simulink model "APS"  (R2020a)
settings: Solver=FixedStepAuto  StartTime=0.0  StopTime=15  FixedStep=0.01  RelTol=1e-3  EnableMultiTasking=on
libraries: embdlinuxlib x3, raspberrypiBasiclib x3
settings Model: SimulationMode=external  Creator=hps  LastModifiedBy=郑亮
settings SolverCC: PositivePriorityOrder=on  AutoInsertRateTranBlk=on
settings DataIOCC: ReturnWorkspaceOutputs=off
settings OptimizationCC: EnhancedBackFolding=on  PassReuseOutputArgsAs=Individual arguments  MaxStackSize=64  OptimizeBlockOrder=speed  DifferentSizesBufferReuse=on  OptimizationCustomize=off  EfficientTunableParamExpr=on
settings DebuggingCC: ParameterTunabilityLossMsg=error  ArithmeticOperatorsInVariantConditions=warning
settings HardwareCC: ProdBitPerPointer=32  ProdBitPerSizeT=32  ProdBitPerPtrDiffT=32  ProdLargestAtomicInteger=Long  ProdLargestAtomicFloat=Double  ProdWordSize=32  ProdHWDeviceType=ARM Compatible->ARM Cortex
settings SFSimCC: MATLABDynamicMemAlloc=off  CustomCodeUndefinedFunction=UseInterfaceOnly
settings RTWCC: SystemTargetFile=ert.tlc  HardwareBoard=Raspberry Pi  TemplateMakefile=ert_default_tmf  GenerateReport=on  Toolchain=GNU GCC Raspberry Pi  BuildConfiguration=Faster Runs  IncludeHyperlinkInReport=on  LaunchReport=on  GenerateTraceInfo=on  GenerateTraceReport=on  GenerateTraceReportSl=on  GenerateTraceReportSf=on  GenerateTraceReportEml=on
settings CodeAppCC: ForceParamTrailComments=on  IgnoreCustomStorageClasses=off  OperatorAnnotations=on  SimulinkDataObjDesc=on  SFDataObjDesc=on  InsertBlockDesc=on
settings ERTTargetCC: SupportContinuousTime=on  SupportVariableSizeSignals=on  ExtModeMexArgs='192.168.43.221' 0 12705

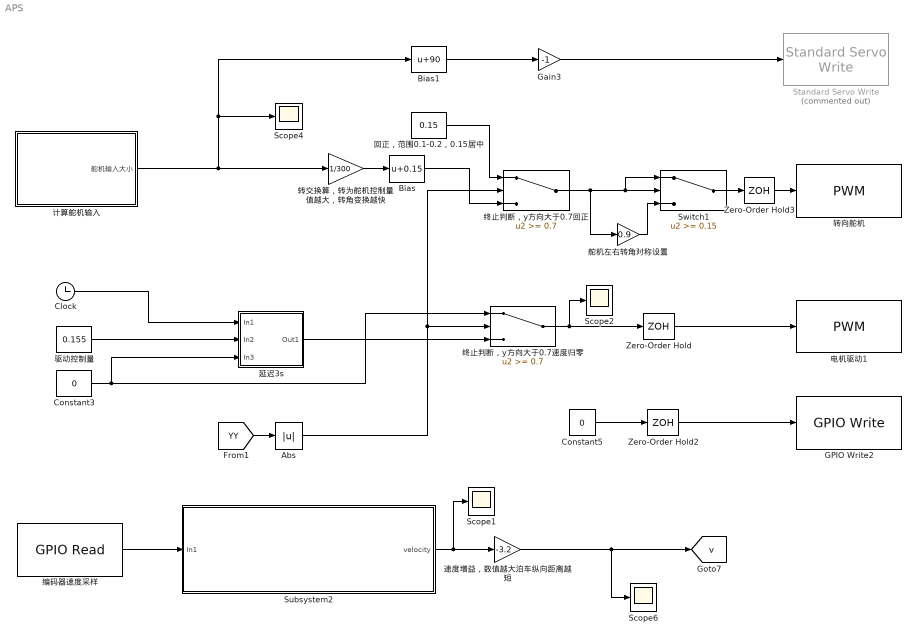
== system APS ==
  Abs : Abs
  Bias : Bias  Bias=0.15
  Bias1 : Bias  Bias=90
  Clock : Clock
  Constant3 : Constant  Value=0
  Constant5 : Constant  Value=0
  GPIO Write2 : embdlinuxlib/GPIO Write  board=Pi 3 Model B+  gpio=27  direction=Output  blockPlatform=Raspberry Pi
      settings: SourceProductBaseCode=SC_BEAGLEBONE_BLUE,RASPPI
  Gain3 : Gain  Gain=-1
  Scope{1..2,4,6} (4 alike) : Scope
  Standard Servo Write : raspberrypiBasiclib/Standard Servo Write  Commented=on  board=Pi 3 Model B+  Pin_=21  MinPulseDuration=1000e-6  MaxPulseDuration=2000e-6  blockPlatform=Raspberry Pi
      settings: SourceProductBaseCode=RASPPI
  Subsystem2 : Subsystem
  Switch1 : Switch  Threshold=0.15
  Zero-Order Hold : ZeroOrderHold  SampleTime=-1
  Zero-Order Hold2 : ZeroOrderHold  SampleTime=-1
  Zero-Order Hold3 : ZeroOrderHold  SampleTime=-1
  回正，范围0.1-0.2，0.15居中 : Constant  Value=0.15
  延迟3s : Subsystem
  电机驱动1 : raspberrypiBasiclib/PWM  board=Pi 3 Model B+  Pin_=17  Frequency=8000  blockPlatform=Raspberry Pi
      settings: SourceProductBaseCode=RASPPI
  终止判断，y方向大于0.7回正 : Switch  Threshold=0.7
  终止判断，y方向大于0.7速度归零 : Switch  Threshold=0.7
  编码器速度采样 : embdlinuxlib/GPIO Read  board=Pi 3 Model B+  gpio=14  internalResistor=Off  sampleTime=0.01  direction=Input  blockPlatform=Raspberry Pi
      settings: SourceProductBaseCode=SC_BEAGLEBONE_BLUE,RASPPI
  舵机左右转角对称设置 : Gain  Gain=0.9
  计算舵机输入 : Subsystem
  "转交换算，转为舵机控制量 值越大，转角变换越快 " : Gain  Gain=1/300
  转向舵机 : raspberrypiBasiclib/PWM  board=Pi 3 Model B  Pin_=21  Frequency=100  blockPlatform=Raspberry Pi
      settings: SourceProductBaseCode=RASPPI
  速度增益，数值越大泊车纵向距离越短 : Gain  Gain=-3.2
  驱动控制量 : Constant  Value=0.155
  tag scope: v=global
  wires:
  Constant3/1 -> 延迟3s/3(In3), 终止判断，y方向大于0.7速度归零/1
  Clock/1 -> 延迟3s/1(In1)
  [YY] -> Abs/1
  Abs/1 -> 终止判断，y方向大于0.7回正/2, 终止判断，y方向大于0.7速度归零/2
  驱动控制量/1 -> 延迟3s/2(In2)
  延迟3s/1(Out1) -> 终止判断，y方向大于0.7速度归零/3
  计算舵机输入/1(舵机输入大小) -> Scope4/1, Bias1/1, "转交换算，转为舵机控制量 值越大，转角变换越快 "/1
  终止判断，y方向大于0.7速度归零/1 -> Zero-Order Hold/1, Scope2/1
  Zero-Order Hold3/1 -> 转向舵机/1
  Constant5/1 -> Zero-Order Hold2/1
  Zero-Order Hold/1 -> 电机驱动1/1
  Zero-Order Hold2/1 -> GPIO Write2/1
  Gain3/1 -> Standard Servo Write/1
  "转交换算，转为舵机控制量 值越大，转角变换越快 "/1 -> Bias/1
  Bias/1 -> 终止判断，y方向大于0.7回正/3
  Bias1/1 -> Gain3/1
  速度增益，数值越大泊车纵向距离越短/1 -> Scope6/1, [v]
  编码器速度采样/1 -> Subsystem2/1(In1)
  Subsystem2/1("velocity ") -> Scope1/1, 速度增益，数值越大泊车纵向距离越短/1
  回正，范围0.1-0.2，0.15居中/1 -> 终止判断，y方向大于0.7回正/1
  终止判断，y方向大于0.7回正/1 -> 舵机左右转角对称设置/1, Switch1/1, Switch1/2
  舵机左右转角对称设置/1 -> Switch1/3
  Switch1/1 -> Zero-Order Hold3/1

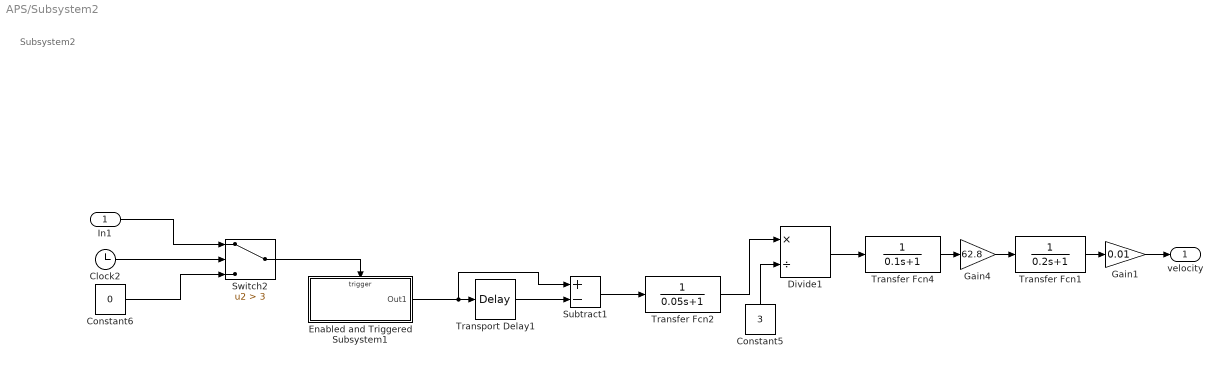
== system APS/Subsystem2 ==
  note: Subsystem2
  In1 : Inport
  Clock2 : Clock
  Constant5 : Constant  Value=3
  Constant6 : Constant  Value=0
  Divide1 : Product  Inputs=*/
  Enabled and Triggered Subsystem1 : Subsystem  TreatAsAtomicUnit=on
  Gain1 : Gain  Gain=0.01
  Gain4 : Gain  Gain=62.8
  Subtract1 : Sum  Inputs=+-
  Switch2 : Switch  Criteria=u2 > Threshold  Threshold=3
  Transfer Fcn1 : TransferFcn  Denominator=[0.2 1]
  Transfer Fcn2 : TransferFcn  Denominator=[0.05 1]
  Transfer Fcn4 : TransferFcn  Denominator=[0.1 1]
  Transport Delay1 : TransportDelay  DelayTime=0.5
  "velocity " : Outport  VectorParamsAs1DForOutWhenUnconnected=off
  wires:
  Constant6/1 -> Switch2/3
  Transport Delay1/1 -> Subtract1/2
  Enabled and Triggered Subsystem1/1(Out1) -> Subtract1/1, Transport Delay1/1
  Switch2/1 -> Enabled and Triggered Subsystem1/Trigger
  Transfer Fcn1/1 -> Gain1/1
  Subtract1/1 -> Transfer Fcn2/1
  Constant5/1 -> Divide1/2
  Clock2/1 -> Switch2/2
  In1/1 -> Switch2/1
  Transfer Fcn2/1 -> Divide1/1
  Gain4/1 -> Transfer Fcn1/1
  Divide1/1 -> Transfer Fcn4/1
  Transfer Fcn4/1 -> Gain4/1
  Gain1/1 -> "velocity "/1

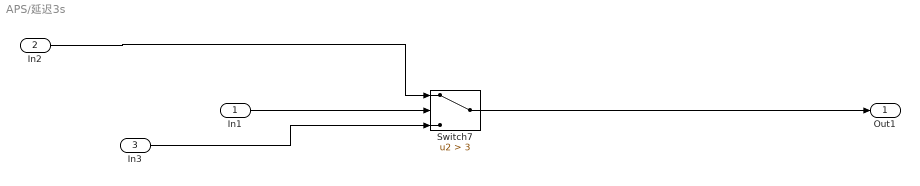
== system APS/延迟3s ==
  In1 : Inport
  In2 : Inport  Port=2
  In3 : Inport  Port=3
  Switch7 : Switch  Criteria=u2 > Threshold  Threshold=3
  Out1 : Outport  VectorParamsAs1DForOutWhenUnconnected=off
  wires:
  In3/1 -> Switch7/3
  In1/1 -> Switch7/2
  In2/1 -> Switch7/1
  Switch7/1 -> Out1/1

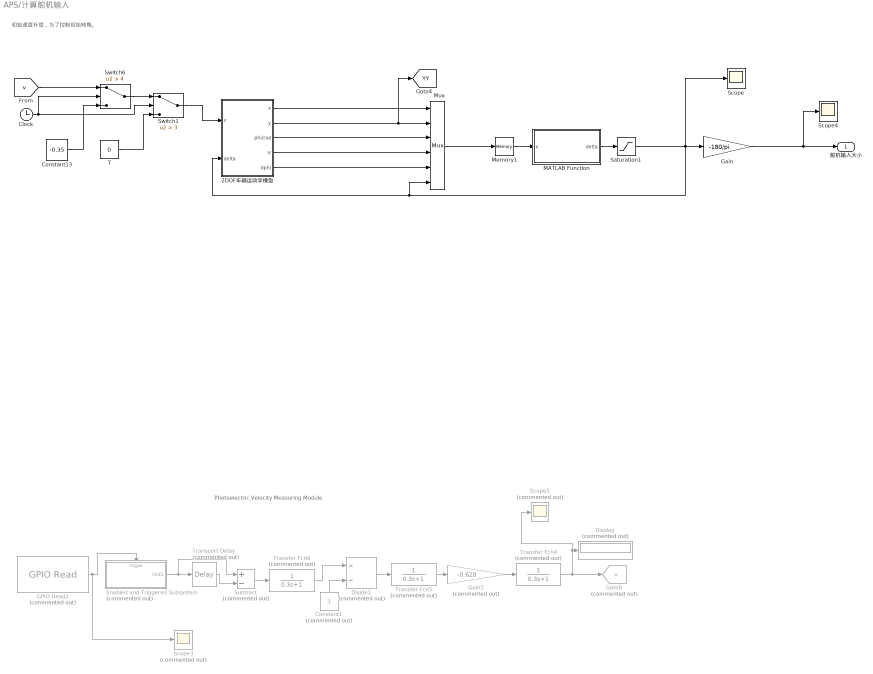
== system APS/计算舵机输入 ==
  note: 初始速度补偿，为了控制初始转角。
  note: Photoelectric Velocity Measuring Module
  2DOF车辆运动学模型 : Subsystem
  Clock : Clock
  Constant1 : Constant  Commented=on  Value=3
  Constant13 : Constant  Value=-0.35
  Display : Display  Commented=on
  Divide1 : Product  Commented=on  Inputs=*/
  Enabled and Triggered Subsystem : Subsystem  Commented=on  TreatAsAtomicUnit=on
  GPIO Read2 : embdlinuxlib/GPIO Read  Commented=on  board=Pi 3 Model B+  gpio=20  internalResistor=Off  sampleTime=0.01  direction=Input  blockPlatform=Raspberry Pi
      settings: SourceProductBaseCode=SC_BEAGLEBONE_BLUE,RASPPI
  Gain : Gain  Gain=-180/pi
  Gain2 : Gain  Commented=on  Gain=-0.628
  Goto8 : Goto  Commented=on  GotoTag=v  TagVisibility=global
  MATLAB Function : MATLAB Function  TreatAsAtomicUnit=on
  Memory1 : Memory
  Mux : Mux  Inputs=6
  Saturation1 : Saturate
  Scope : Scope
  Scope3 : Scope  Commented=on
  Scope4 : Scope
  Scope5 : Scope  Commented=on
  Subtract : Sum  Commented=on  Inputs=+-
  Switch1 : Switch  Criteria=u2 > Threshold  Threshold=3
  Switch6 : Switch  Criteria=u2 > Threshold  Threshold=4
  T : Constant  Value=0
  Transfer Fcn4 : TransferFcn  Commented=on  Denominator=[0.3 1]
  Transfer Fcn5 : TransferFcn  Commented=on  Denominator=[0.3 1]
  Transfer Fcn6 : TransferFcn  Commented=on  Denominator=[0.3 1]
  Transport Delay : TransportDelay  Commented=on  DelayTime=0.5
  舵机输入大小 : Outport  VectorParamsAs1DForOutWhenUnconnected=off
  tag scope: YY=global
  wires:
  Memory1/1 -> MATLAB Function/1(x)
  MATLAB Function/1(delta) -> Saturation1/1
  2DOF车辆运动学模型/5(dphi) -> Mux/5
  Switch1/1 -> 2DOF车辆运动学模型/1(v)
  2DOF车辆运动学模型/4(V) -> Mux/4
  2DOF车辆运动学模型/1(x) -> Mux/1
  2DOF车辆运动学模型/3(phi/rad) -> Mux/3
  Saturation1/1 -> Scope/1, Gain/1, Mux/6, 2DOF车辆运动学模型/2(delta)
  [v] -> Switch6/1
  2DOF车辆运动学模型/2(y) -> Mux/2, [YY]
  Mux/1 -> Memory1/1
  Transport Delay/1 -> Subtract/2
  Enabled and Triggered Subsystem/1(Out1) -> Transport Delay/1, Subtract/1
  Transfer Fcn4/1 -> Goto8/1, Scope5/1, Display/1
  Transfer Fcn5/1 -> Gain2/1
  Gain2/1 -> Transfer Fcn4/1
  Transfer Fcn6/1 -> Divide1/1
  Constant1/1 -> Divide1/2
  Subtract/1 -> Transfer Fcn6/1
  Divide1/1 -> Transfer Fcn5/1
  GPIO Read2/1 -> Scope3/1, Enabled and Triggered Subsystem/Trigger
  Gain/1 -> Scope4/1, 舵机输入大小/1
  Switch6/1 -> Switch1/1
  T/1 -> Switch1/3
  Constant13/1 -> Switch6/3
  Clock/1 -> Switch6/2, Switch1/2

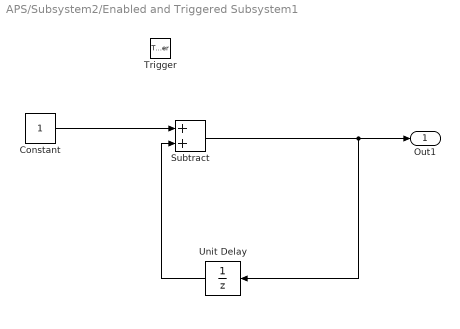
== system APS/Subsystem2/Enabled and Triggered Subsystem1 ==
  Trigger : TriggerPort  TriggerType=falling  VariantControl=Variant
  Constant : Constant
  Subtract : Sum
  Unit Delay : UnitDelay  SampleTime=-1  HasFrameUpgradeWarning=on
  Out1 : Outport  VectorParamsAs1DForOutWhenUnconnected=off
  wires:
  Constant/1 -> Subtract/1
  Subtract/1 -> Unit Delay/1, Out1/1
  Unit Delay/1 -> Subtract/2

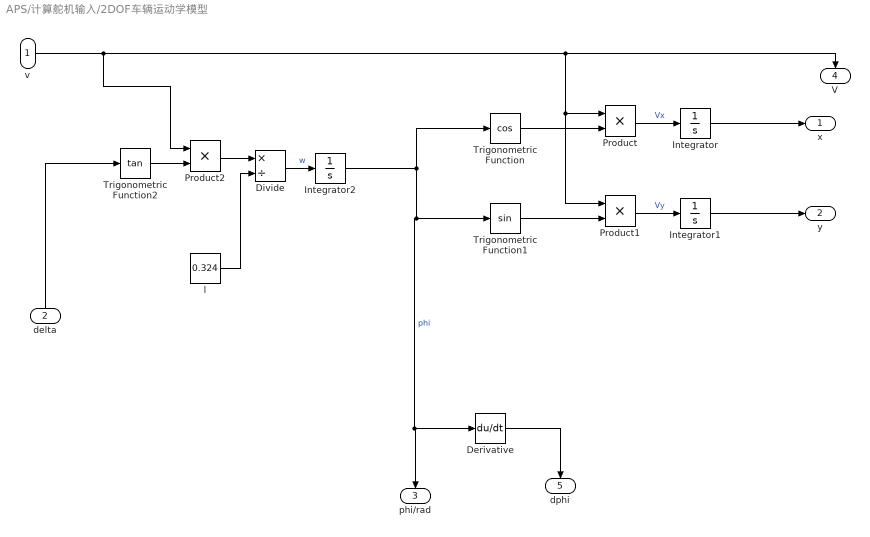
== system APS/计算舵机输入/2DOF车辆运动学模型 ==
  v : Inport
  delta : Inport  Port=2
  Derivative : Derivative
  Divide : Product  Inputs=*/
  Integrator : Integrator
  Integrator1 : Integrator
  Integrator2 : Integrator
  Product : Product
  Product1 : Product
  Product2 : Product
  Trigonometric Function : Trigonometry  Operator=cos
  Trigonometric Function1 : Trigonometry
  Trigonometric Function2 : Trigonometry  Operator=tan
  l : Constant  Value=0.324
  x : Outport  VectorParamsAs1DForOutWhenUnconnected=off
  y : Outport  Port=2  VectorParamsAs1DForOutWhenUnconnected=off
  phi/rad : Outport  Port=3  VectorParamsAs1DForOutWhenUnconnected=off
  V : Outport  Port=4  VectorParamsAs1DForOutWhenUnconnected=off
  dphi : Outport  Port=5  VectorParamsAs1DForOutWhenUnconnected=off
  wires:
  Derivative/1 -> dphi/1
  v/1 -> Product2/1, Product/1, Product1/1, V/1
  delta/1 -> Trigonometric Function2/1
  Integrator/1 -> x/1
  Integrator2/1 -> phi/rad/1, Derivative/1, Trigonometric Function1/1, Trigonometric Function/1  "phi"
  Integrator1/1 -> y/1
  Product1/1 -> Integrator1/1  "Vy"
  Trigonometric Function1/1 -> Product1/2
  Divide/1 -> Integrator2/1  "w"
  Product2/1 -> Divide/1
  Trigonometric Function/1 -> Product/2
  Trigonometric Function2/1 -> Product2/2
  l/1 -> Divide/2
  Product/1 -> Integrator/1  "Vx"

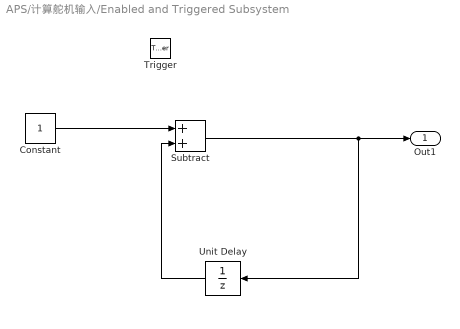
== system APS/计算舵机输入/Enabled and Triggered Subsystem ==
  Trigger : TriggerPort  TriggerType=falling  VariantControl=Variant
  Constant : Constant
  Subtract : Sum
  Unit Delay : UnitDelay  SampleTime=-1  HasFrameUpgradeWarning=on
  Out1 : Outport  VectorParamsAs1DForOutWhenUnconnected=off
  wires:
  Constant/1 -> Subtract/1
  Subtract/1 -> Unit Delay/1, Out1/1
  Unit Delay/1 -> Subtract/2

== matlab function APS/计算舵机输入/MATLAB Function ==
  data: x input; delta output
function delta = fcn(x)

    Nx = 3;%状态量的个数
    Nu = 2;%控制量的个数
    Ny = 2; %输出量的个数
    Np = 20;%预测步长
    Nc = 5;%控制步长
    Row = 1000;%松弛因子

    u = zeros(6,1);
    u = x;
    U = [0;u(6)];
    
    t_d =u(3);
    vd1=u(4);
    vd2=u(6); 
    
    kesi=zeros(Nx+Nu,1);  
    kesi(1)=u(1);
    kesi(2)=u(2);
    kesi(3)=u(3);   % 角度单位要一致！！！！！    
    kesi(4)=U(1);
    kesi(5)=U(2); 

    T=0.04;
    L = 0.324;
    
    u_piao=zeros(Nu,1);
    
    Q = zeros(2*Np,2*Np);
   for i=1:1:2*Np
       for j=1:1:2*Np
           if i==j
               if mod(i,2)==0
                   Q(i,j) = 1;
               else
                   Q(i,j) = 10;
               end
           else 
               Q(i,j)= 0;               
           end
       end 
   end 

    R = 10*eye(Nu*Nc);
    
    a=[1    0   -vd1*sin(t_d)*T;
       0    1   vd1*cos(t_d)*T;
       0    0   1;];
    b=[cos(t_d)*T            0;
       sin(t_d)*T            0;
       tan(vd2)*T/L      vd1*T/(cos(vd2)^2);];

    A = zeros(5,5);
    B = zeros(5,2);
    A(1:3,1:3)=a;
    A(1:3,4:5)=b;
    A(4:5,4:5)=eye(Nu);
    
    B(1:3,1:2)=b;
    B(4:5,1:2)=eye(Nu);

    C=[0 1 0 0 0;0 0 1 0 0;];

%% 计算偏差
    d_k=zeros(Nx,1);%计算偏差
    state_k1=zeros(Nx,1);%预测的下一时刻状态量，用于计算偏差
    state_k1(1,1)=u(1)+T*u(4)*cos(t_d);
    state_k1(2,1)=u(2)+T*u(4)*sin(t_d);
    state_k1(3,1)=t_d+T*u(5);
    d_k=state_k1-a*kesi(1:3,1)-b*kesi(4:5,1);
    d_piao_k=zeros(Nx+Nu,1);
    d_piao_k(1:3,1)=d_k;
    d_piao_k(4,1)=0;
    d_piao_k(5,1)=0;
    
    PHI = zeros(100,1);
    GAMMA = zeros(40,100);

    for p=1:1:Np
        PHI((5*(p-1)+1):(5*p),1)=d_piao_k;
        for q=1:1:Np
            if q<=p
                GAMMA((2*(p-1)+1):2*p,(5*(q-1)+1):5*q)=C*A^(p-q);
            else 
                GAMMA((2*(p-1)+1):2*p,(5*(q-1)+1):5*q)=zeros(Ny,Nx+Nu);
            end 
        end
    end
 
    PSI = zeros(40,5);
    THETA = zeros(40,10);
    for j=1:1:Np
       PSI((2*(j-1)+1):2*j,1:5)=C*A^j;
        for k=1:1:Nc
            if k<=j
                THETA((2*(j-1)+1):2*j,(2*(k-1)+1):2*k) = C*A^(j-k)*B;
            else 
                THETA((2*(j-1)+1):2*j,(2*(k-1)+1):2*k) = zeros(Ny,Nu);
            end
        end
    end    

    H = zeros(10,10);
    H(1:10,1:10)=THETA'*Q*THETA+R;
%     H(1:10,11)=zeros(Nu*Nc,1);
%     H(11,1:10)=zeros(1,Nu*Nc);
%     H(11,11)=Row;
        
%% 参考轨迹生成
    X_predict=zeros(Np,1);%用于保存预测时域内的纵向位置信息，这是计算期望轨迹的基础
    phi_ref=zeros(Np,1);%用于保存预测时域内的期望轨迹
    Y_ref=zeros(Np,1);%用于保存预测时域内的期望轨迹    
    Yita_ref=zeros(2*Np,1);
    error_1=zeros(Nx*Np,1);
    for p=1:1:Np
    %x=8 y=2.5
          X_predict(p,1)=u(1)+u(4)*cos(t_d)*p*T;
%           Y_ref(p,1)= 0.2;
%           phi_ref(p,1)=0;       
          Y_ref(p,1)=0.7/2*X_predict(p,1)-(-0.7/(2*pi))*sin((2*pi*X_predict(p,1))/(-2));
          phi_ref(p,1)=atan(0.7/2-(-0.7/(2*pi))*cos(2*pi*X_predict(p,1)/(-2))*2*pi/(-2)); 
          if Y_ref(p,1)<-0.7
             Y_ref(p,1)= -0.7;
             phi_ref(p,1) = 0;
          end
          Yita_ref((2*(p-1)+1):2*p,1)=[Y_ref(p,1);phi_ref(p,1)];
    end
    
    error_1=Yita_ref-PSI*kesi-GAMMA*PHI; %求偏差
    f=zeros(1,10);
%     f(1,1:10)=-2*error_1'*Q*THETA;
    f(1,1:10)=-2*error_1'*Q*THETA;
%     f(1,11)=0;
    f = f';
    
 %% 以下为约束生成区域
 %不等式约束
    A_t=zeros(Nc,Nc);
    for p=1:1:Nc
        for q=1:1:Nc
            if q<=p 
                A_t(p,q)=1;
            else 
                A_t(p,q)=0;
            end
        end 
    end 
    A_I=kron(A_t,eye(Nu));
    Ut=kron(ones(Nc,1),U);
    umin=[-0.2;-0.436];%维数与控制变量的个数相同
    umax=[0.2;0.436];
    delta_umin=[-0.05;-0.0436;];
    delta_umax=[0.05;0.0436];
    Umin=kron(ones(Nc,1),umin);
    Umax=kron(ones(Nc,1),umax);
    delta_Umin=kron(ones(Nc,1),delta_umin);
    delta_Umax=kron(ones(Nc,1),delta_umax);
    
%    A_cons = zeros(20,10);
%    b_cons = zeros(20,1);
%     A_cons=[A_I zeros(Nu*Nc,1);-A_I zeros(Nu*Nc,1)];
%     b_cons=[Umax-Ut;-Umin+Ut]; 

    A_cons=[A_I;-A_I;eye(10);-eye(10)];
    b_cons=[Umin-Ut;-Umax+Ut;delta_Umin;-delta_Umax]; 
    
    Aeq = [];
    beq = zeros(0,1);
    [L,p] = chol(H,'lower');
    Linv = inv(L);
    for p=1:1:10
        for q=1:1:10
            if q>p 
                Linv(p,q)=0;
            end
        end 
    end 
    opt = mpcqpsolverOptions;
    iA0 = false(size(b_cons));
    [X] = mpcqpsolver(Linv,f,A_cons,b_cons,Aeq,beq,iA0,opt);
    
    delta = X(2,1)+u(6);
